simulink model "check_modelcompare_heaviside"  (R2018b)
settings: configuration reference "Physics" (kept outside this file)
undefined symbols (not defined in the file or in its folder): brake_param, veh_param, x0_positionstates
libraries: simulink x4
settings Model: DataDictionary=check_modelcompare.sldd  OrderedModelArguments=off  Creator=wischnewski  LastModifiedBy=ga25xiw

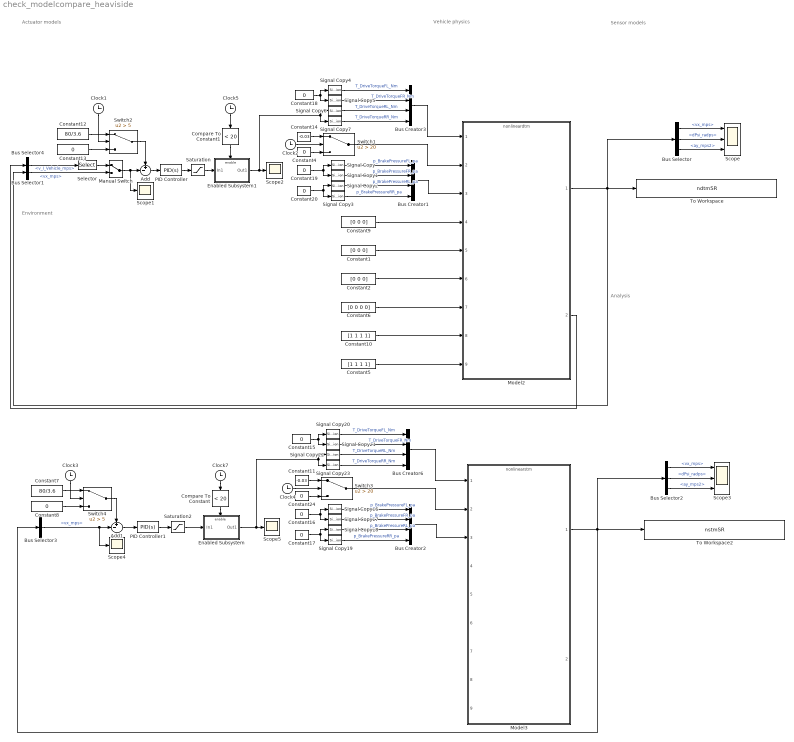
== system check_modelcompare_heaviside ==
  note: Actuator models
  note: Vehicle physics
  note: Environment
  note: Analysis
  note: Sensor models
  Add : Sum  Inputs=+-|
  Add1 : Sum  Inputs=+-|
  Bus Creator1 : BusCreator  Inputs=4  OutDataTypeStr=Bus: BrakePressure_Pa
  Bus Creator2 : BusCreator  Inputs=4  OutDataTypeStr=Bus: BrakePressure_Pa
  Bus Creator3 : BusCreator  Inputs=4  OutDataTypeStr=Bus: DriveTorque_Nm
  Bus Creator6 : BusCreator  Inputs=4  OutDataTypeStr=Bus: DriveTorque_Nm
  Bus Selector : BusSelector  OutputSignals=vx_mps,dPsi_radps,ay_mps2
  Bus Selector1 : BusSelector  OutputSignals=vx_mps
  Bus Selector2 : BusSelector  OutputSignals=vx_mps,dPsi_radps,ay_mps2
  Bus Selector3 : BusSelector  OutputSignals=vx_mps
  Bus Selector4 : BusSelector  OutputSignals=Vehicle.v_I_Vehicle_mps
  Clock{1..5,7} (6 alike) : Clock
  Compare To Constant : simulink/Logic and Bit Operations/Compare To Constant  relop=<  const=20  OutDataTypeStr=boolean
  Compare To Constant1 : simulink/Logic and Bit Operations/Compare To Constant  relop=<  const=20  OutDataTypeStr=boolean
  Constant1 : Constant  Value=[0 0 0]
  Constant10 : Constant  Value=[1 1 1 1]
  Constant11 : Constant  Value=-0.03
  Constant12 : Constant  Value=80/3.6
  Constant{4,8,13,15..20,24} (10 alike) : Constant  Value=0
  Constant14 : Constant  Value=-0.03
  Constant2 : Constant  Value=[0 0 0]
  Constant5 : Constant  Value=[1 1 1 1]
  Constant6 : Constant  Value=[0 0 0 0]
  Constant7 : Constant  Value=80/3.6
  Constant9 : Constant  Value=[0 0 0]
  Enabled Subsystem : Subsystem  TreatAsAtomicUnit=on
  Enabled Subsystem1 : Subsystem  TreatAsAtomicUnit=on
  Manual Switch : ManualSwitch
  Model2 : ModelReference  ModelNameDialog=nonlineardtm  ParameterArgumentNames=x0_vehiclepose  ParameterArgumentValues=[0,0,-pi/2]  UsingDefaultArgumentValue=0  SimulationMode=Normal  ModelReferenceVersion=1.633
  Model3 : ModelReference  ModelNameDialog=nonlinearstm.slx  ParameterArgumentNames=brake_param,veh_param,x0_positionstates  ParameterArgumentValues=brake_param,veh_param,[0,0,-pi/2]  UsingDefaultArgumentValue=0,0,0  SimulationMode=Normal  ModelReferenceVersion=1.335
  PID Controller : simulink/Continuous/PID Controller  Controller=PID  Form=Parallel  TimeDomain=Continuous-time  SampleTime=-1  IntegratorMethod=Forward Euler  FilterMethod=Forward Euler  ControllerParametersSource=internal  P=1000  I=1  D=0  UseFilter=on  N=100  TunerSelectOption=Transfer Function Based (PID Tuner App)  InitialConditionSource=internal  InitialConditionForIntegrator=0  InitialConditionForFilter=0  DifferentiatorICPrevScaledInput=0  ExternalReset=none  TrackingMode=off  Kt=1  LimitOutput=off  UpperSaturationLimit=inf  LowerSaturationLimit=-inf  LinearizeAsGain=on  AntiWindupMode=none  Kb=1  POutMin=[]  POutMax=[]  IOutMin=[]  IOutMax=[]  DOutMin=[]  DOutMax=[]  NOutMin=[]  NOutMax=[]  SumOutMin=[]  SumOutMax=[]  SaturationOutMin=[]  SaturationOutMax=[]  PParamMin=[]  PParamMax=[]  IParamMin=[]  IParamMax=[]  DParamMin=[]  DParamMax=[]  NParamMin=[]  NParamMax=[]  KbParamMin=[]  KbParamMax=[]  KtParamMin=[]  KtParamMax=[]  KbOutMin=[]  KbOutMax=[]  KtOutMin=[]  KtOutMax=[]  IntegratorOutMin=[]  IntegratorOutMax=[]  FilterOutMin=[]  FilterOutMax=[]  SumI1OutMin=[]  SumI1OutMax=[]  SumI2OutMin=[]  SumI2OutMax=[]  SumI3OutMin=[]  SumI3OutMax=[]  SumI4OutMin=[]  SumI4OutMax=[]  SumDOutMin=[]  SumDOutMax=[]  DifferentiatorOutMin=[]  DifferentiatorOutMax=[]  FilterDiffOutCoefMin=[]  FilterDiffOutCoefMax=[]  ReciprocalOutMin=[]  ReciprocalOutMax=[]  SumDenOutMin=[]  SumDenOutMax=[]  SumNumOutMin=[]  SumNumOutMax=[]  DivideOutMin=[]  DivideOutMax=[]  IntegratorContinuousStateAttributes=''  IntegratorStateMustResolveToSignalObject=off  IntegratorRTWStateStorageClass=Auto  FilterContinuousStateAttributes=''  FilterStateMustResolveToSignalObject=off  FilterRTWStateStorageClass=Auto  ParallelPVariant=InternalParameters  IdealPVariant=Disabled  IVariant=InternalParameters  DVariant=InternalParameters  IntegratorVariant=Continuous  SatVariant=Disabled  AWVariant=Passthrough  PCopyVariant=Disabled  TRVariant=Disabled  FdbkBlocksVariant=Forward  IdealPFdbkVariant=Disabled  SatFdbkVariant=Disabled  DerivativeFilterVariant=ContFilter  NVariant=InternalParameters  NCopyVariant=Disabled  FilterICVariant=InternalICsFilter  IntegratorICVariant=InternalICs  ExternalResetVariant=Disabled  TRSumVariant=Passthrough  SumFdbkVariant=Disabled  SumVariant=Sum_PID
  PID Controller1 : simulink/Continuous/PID Controller  Controller=PID  Form=Parallel  TimeDomain=Continuous-time  SampleTime=-1  IntegratorMethod=Forward Euler  FilterMethod=Forward Euler  ControllerParametersSource=internal  P=1000  I=0.5  D=0  UseFilter=on  N=100  TunerSelectOption=Transfer Function Based (PID Tuner App)  InitialConditionSource=internal  InitialConditionForIntegrator=0  InitialConditionForFilter=0  DifferentiatorICPrevScaledInput=0  ExternalReset=none  TrackingMode=off  Kt=1  LimitOutput=off  UpperSaturationLimit=inf  LowerSaturationLimit=-inf  LinearizeAsGain=on  AntiWindupMode=none  Kb=1  POutMin=[]  POutMax=[]  IOutMin=[]  IOutMax=[]  DOutMin=[]  DOutMax=[]  NOutMin=[]  NOutMax=[]  SumOutMin=[]  SumOutMax=[]  SaturationOutMin=[]  SaturationOutMax=[]  PParamMin=[]  PParamMax=[]  IParamMin=[]  IParamMax=[]  DParamMin=[]  DParamMax=[]  NParamMin=[]  NParamMax=[]  KbParamMin=[]  KbParamMax=[]  KtParamMin=[]  KtParamMax=[]  KbOutMin=[]  KbOutMax=[]  KtOutMin=[]  KtOutMax=[]  IntegratorOutMin=[]  IntegratorOutMax=[]  FilterOutMin=[]  FilterOutMax=[]  SumI1OutMin=[]  SumI1OutMax=[]  SumI2OutMin=[]  SumI2OutMax=[]  SumI3OutMin=[]  SumI3OutMax=[]  SumI4OutMin=[]  SumI4OutMax=[]  SumDOutMin=[]  SumDOutMax=[]  DifferentiatorOutMin=[]  DifferentiatorOutMax=[]  FilterDiffOutCoefMin=[]  FilterDiffOutCoefMax=[]  ReciprocalOutMin=[]  ReciprocalOutMax=[]  SumDenOutMin=[]  SumDenOutMax=[]  SumNumOutMin=[]  SumNumOutMax=[]  DivideOutMin=[]  DivideOutMax=[]  IntegratorContinuousStateAttributes=''  IntegratorStateMustResolveToSignalObject=off  IntegratorRTWStateStorageClass=Auto  FilterContinuousStateAttributes=''  FilterStateMustResolveToSignalObject=off  FilterRTWStateStorageClass=Auto  ParallelPVariant=InternalParameters  IdealPVariant=Disabled  IVariant=InternalParameters  DVariant=InternalParameters  IntegratorVariant=Continuous  SatVariant=Disabled  AWVariant=Passthrough  PCopyVariant=Disabled  TRVariant=Disabled  FdbkBlocksVariant=Forward  IdealPFdbkVariant=Disabled  SatFdbkVariant=Disabled  DerivativeFilterVariant=ContFilter  NVariant=InternalParameters  NCopyVariant=Disabled  FilterICVariant=InternalICsFilter  IntegratorICVariant=InternalICs  ExternalResetVariant=Disabled  TRSumVariant=Passthrough  SumFdbkVariant=Disabled  SumVariant=Sum_PID
  Saturation : Saturate  UpperLimit=1250  LowerLimit=0
  Saturation2 : Saturate  UpperLimit=1250  LowerLimit=0
  Scope : Scope  NumInputPorts=3
  Scope{1..2,4..5} (4 alike) : Scope
  Scope3 : Scope  NumInputPorts=3
  Selector : Selector  InputPortWidth=3  IndexOptions=Index vector (dialog)  Indices=1  OutputSizes=1
  Signal Copy{,1..7,16..23} (16 alike) : SignalConversion  OverrideOpt=off
  Switch1 : Switch  Criteria=u2 > Threshold  Threshold=20
  Switch2 : Switch  Criteria=u2 > Threshold  Threshold=5
  Switch3 : Switch  Criteria=u2 > Threshold  Threshold=20
  Switch4 : Switch  Criteria=u2 > Threshold  Threshold=5
  To Workspace : ToWorkspace  VariableName=ndtmSR  SaveFormat=Timeseries  SampleTime=-1
  To Workspace2 : ToWorkspace  VariableName=nstmSR  SaveFormat=Timeseries  SampleTime=-1
  wires:
  Bus Selector/1 -> Scope/1  "<vx_mps>"
  Bus Selector/2 -> Scope/2  "<dPsi_radps>"
  Bus Selector/3 -> Scope/3  "<ay_mps2>"
  Constant9/1 -> Model2/4
  Constant1/1 -> Model2/5
  Constant2/1 -> Model2/6
  Constant5/1 -> Model2/9
  Model2/1 -> Bus Selector1/1, Bus Selector/1, To Workspace/1
  Constant6/1 -> Model2/7
  Manual Switch/1 -> Scope1/1, Add/2
  PID Controller/1 -> Saturation/1
  Add/1 -> PID Controller/1
  Constant12/1 -> Switch2/1
  Constant13/1 -> Switch2/3
  Clock1/1 -> Switch2/2
  Switch2/1 -> Add/1
  Constant10/1 -> Model2/8
  Constant4/1 -> Switch1/3
  Constant14/1 -> Switch1/1
  Clock2/1 -> Switch1/2
  Switch1/1 -> Model2/2
  Model3/1 -> Bus Selector2/1, To Workspace2/1, Bus Selector3/1
  Constant7/1 -> Switch4/1
  Clock3/1 -> Switch4/2
  Add1/1 -> PID Controller1/1
  Bus Selector2/2 -> Scope3/2  "<dPsi_radps>"
  Switch4/1 -> Add1/1
  Bus Selector2/3 -> Scope3/3  "<ay_mps2>"
  Bus Selector3/1 -> Scope4/1, Add1/2  "<vx_mps>"
  Bus Selector2/1 -> Scope3/1  "<vx_mps>"
  Constant8/1 -> Switch4/3
  PID Controller1/1 -> Saturation2/1
  Saturation2/1 -> Enabled Subsystem/1(In1)
  Clock7/1 -> Compare To Constant/1
  Compare To Constant/1 -> Enabled Subsystem/Enable
  Clock5/1 -> Compare To Constant1/1
  Saturation/1 -> Enabled Subsystem1/1(In1)
  Compare To Constant1/1 -> Enabled Subsystem1/Enable
  Model2/2 -> Bus Selector4/1
  Bus Selector4/1 -> Selector/1  "<v_I_Vehicle_mps>"
  Bus Selector1/1 -> Manual Switch/2  "<vx_mps>"
  Selector/1 -> Manual Switch/1
  Signal Copy5/1 -> Bus Creator3/2  "T_DriveTorqueFR_Nm"
  Signal Copy3/1 -> Bus Creator1/4  "p_BrakePressureRR_pa"
  Signal Copy2/1 -> Bus Creator1/3  "p_BrakePressureRL_pa"
  Constant20/1 -> Signal Copy3/1, Signal Copy2/1
  Enabled Subsystem1/1(Out1) -> Signal Copy7/1, Signal Copy6/1, Scope2/1
  Constant18/1 -> Signal Copy4/1, Signal Copy5/1
  Signal Copy6/1 -> Bus Creator3/3  "T_DriveTorqueRL_Nm"
  Constant19/1 -> Signal Copy1/1, Signal Copy/1
  Signal Copy4/1 -> Bus Creator3/1  "T_DriveTorqueFL_Nm"
  Signal Copy7/1 -> Bus Creator3/4  "T_DriveTorqueRR_Nm"
  Bus Creator1/1 -> Model2/3
  Bus Creator3/1 -> Model2/1
  Signal Copy/1 -> Bus Creator1/1  "p_BrakePressureFL_pa"
  Signal Copy1/1 -> Bus Creator1/2  "p_BrakePressureFR_pa"
  Constant24/1 -> Switch3/3
  Clock4/1 -> Switch3/2
  Constant11/1 -> Switch3/1
  Signal Copy16/1 -> Bus Creator2/1  "p_BrakePressureFL_pa"
  Bus Creator6/1 -> Model3/1
  Signal Copy23/1 -> Bus Creator6/4  "T_DriveTorqueRR_Nm"
  Signal Copy20/1 -> Bus Creator6/1  "T_DriveTorqueFL_Nm"
  Constant15/1 -> Signal Copy20/1, Signal Copy21/1
  Constant16/1 -> Signal Copy17/1, Signal Copy16/1
  Signal Copy22/1 -> Bus Creator6/3  "T_DriveTorqueRL_Nm"
  Signal Copy21/1 -> Bus Creator6/2  "T_DriveTorqueFR_Nm"
  Switch3/1 -> Model3/2
  Signal Copy19/1 -> Bus Creator2/4  "p_BrakePressureRR_pa"
  Signal Copy17/1 -> Bus Creator2/2  "p_BrakePressureFR_pa"
  Constant17/1 -> Signal Copy19/1, Signal Copy18/1
  Signal Copy18/1 -> Bus Creator2/3  "p_BrakePressureRL_pa"
  Enabled Subsystem/1(Out1) -> Signal Copy23/1, Signal Copy22/1, Scope5/1
  Bus Creator2/1 -> Model3/3

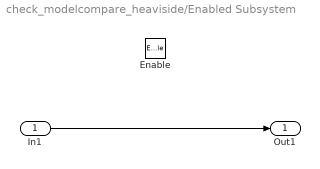
== system check_modelcompare_heaviside/Enabled Subsystem ==
  In1 : Inport
  Enable : EnablePort
  Out1 : Outport
  wires:
  In1/1 -> Out1/1

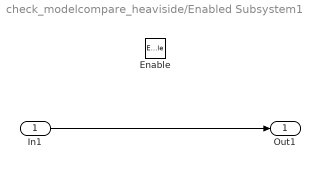
== system check_modelcompare_heaviside/Enabled Subsystem1 ==
  In1 : Inport
  Enable : EnablePort
  Out1 : Outport
  wires:
  In1/1 -> Out1/1
